simulink model "sim_IDmodel_3pools"  (Simulink 6.3)
settings: Solver=ode45  StartTime=0.0  StopTime=100  RelTol=1e-7
values from neighbouring files (symbols this model uses):
  Ad = [1 5 1]    [PI_mixed_3pools.m]
  dec_DD = 1*[0.8 0.9]    [PI_mixed_3pools.m]
  dec_LU = 1*[1 1]    [PI_mixed_3pools.m]
  t_step1 = 1    [PI_mixed_3pools.m]
  t_step2 = 50    [PI_mixed_3pools.m]
  t_step3 = 100    [PI_mixed_3pools.m]
  tau = [1 1 1]    [PI_mixed_3pools.m]
undefined symbols (not defined in the file or in its folder): K1, K1b, K2
libraries: cstblocks x9
settings Model: LastModifiedBy=IRMOPerm  StrictBusMsg=None
settings DataIOCC: SignalLoggingName=sigsOut
settings DebuggingCC: SolverPrmCheckMsg=none
settings HardwareCC: TargetUnknown=on
settings GRTTargetCC: ModelReferenceCompliant=off  MatFileLogging=off

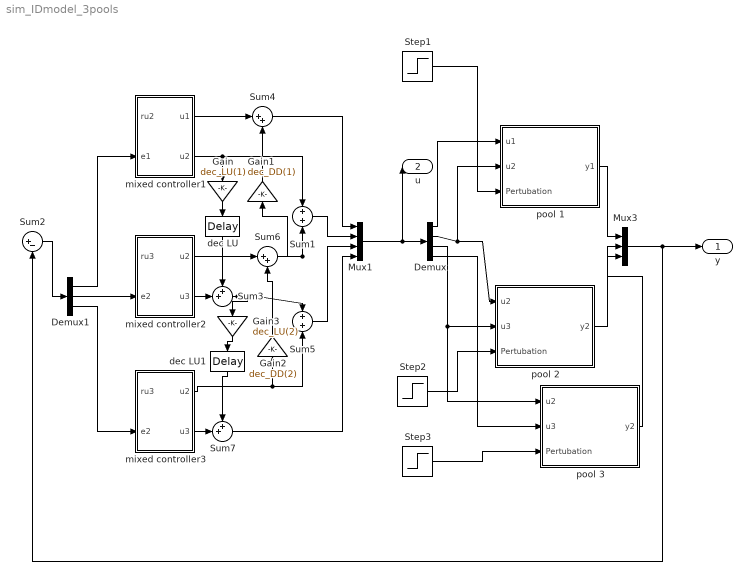
== system sim_IDmodel_3pools ==
  Demux : Demux
  Demux1 : Demux  Outputs=3
  Gain : Gain  Orientation=down  Gain=dec_LU(1)
  Gain1 : Gain  Orientation=up  Gain=dec_DD(1)
  Gain2 : Gain  Orientation=up  Gain=dec_DD(2)
  Gain3 : Gain  Orientation=down  Gain=dec_LU(2)
  Mux1 : Mux
  Mux3 : Mux  Inputs=3
  Step1 : Step  Time=t_step1  SampleTime=0
  Step2 : Step  Time=t_step2  SampleTime=0
  Step3 : Step  Time=t_step3  SampleTime=0
  Sum1 : Sum  SaturateOnIntegerOverflow=on  InputSameDT=on
  Sum2 : Sum  Inputs=|+-  SaturateOnIntegerOverflow=on  InputSameDT=on
  Sum3 : Sum  Inputs=++|  SaturateOnIntegerOverflow=on  InputSameDT=on
  Sum4 : Sum  Inputs=|++  SaturateOnIntegerOverflow=on  InputSameDT=on
  Sum5 : Sum  SaturateOnIntegerOverflow=on  InputSameDT=on
  Sum6 : Sum  Inputs=|++  SaturateOnIntegerOverflow=on  InputSameDT=on
  Sum7 : Sum  Inputs=++|  SaturateOnIntegerOverflow=on  InputSameDT=on
  dec LU : TransportDelay  Orientation=down  DelayTime=tau(2)
  dec LU1 : TransportDelay  Orientation=down  DelayTime=tau(3)
  mixed controller1 : Subsystem
  mixed controller2 : Subsystem
  mixed controller3 : Subsystem
  pool 1 : Subsystem
  pool 2 : Subsystem
  pool 3 : Subsystem
  y : Outport
  u : Outport  Port=2
  wires:
  Mux1/1 -> u/1, Demux/1
  Sum2/1 -> Demux1/1
  Step1/1 -> pool 1/3(Pertubation)
  Demux/2 -> pool 1/2(u2), pool 2/1("u2 ")
  pool 1/1(y1) -> Mux3/1
  pool 2/1(y2) -> Mux3/2
  Demux/1 -> pool 1/1("u1 ")
  Demux/3 -> pool 2/2(u3), pool 3/1("u2 ")
  Mux3/1 -> Sum2/2, y/1
  Demux1/2 -> mixed controller2/2(e2)
  Demux1/1 -> mixed controller1/2(e1)
  mixed controller1/2(u2) -> Sum1/1, Gain/1
  mixed controller2/1(u2) -> Sum6/1
  dec LU/1 -> Sum3/1
  mixed controller2/2(u3) -> Sum3/2
  Gain/1 -> dec LU/1
  Gain1/1 -> Sum4/2
  mixed controller1/1(u1) -> Sum4/1
  Sum4/1 -> Mux1/1
  Sum1/1 -> Mux1/2
  Step2/1 -> pool 2/3(Pertubation)
  Demux1/3 -> mixed controller3/2(e2)
  Sum3/1 -> Gain3/1, Sum5/1
  Gain2/1 -> Sum6/2
  mixed controller3/1(u2) -> Sum5/2, Gain2/1
  dec LU1/1 -> Sum7/1
  Gain3/1 -> dec LU1/1
  Sum7/1 -> Mux1/4
  mixed controller3/2(u3) -> Sum7/2
  Sum6/1 -> Sum1/2, Gain1/1
  Sum5/1 -> Mux1/3
  Demux/4 -> pool 3/2(u3)
  Step3/1 -> pool 3/3(Pertubation)
  pool 3/1(y2) -> Mux3/3

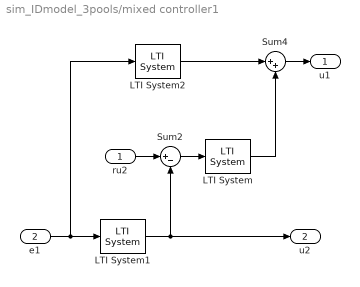
== system sim_IDmodel_3pools/mixed controller1 ==
  ru2 : Inport
  e1 : Inport  Port=2
  LTI System : cstblocks/LTI System  sys=K1b(1)  IC=[]
  LTI System1 : cstblocks/LTI System  sys=K2(1)  IC=[]
  LTI System2 : cstblocks/LTI System  sys=K1(1)  IC=[]
  Sum2 : Sum  Inputs=|+-  SaturateOnIntegerOverflow=on  InputSameDT=on
  Sum4 : Sum  Inputs=|++  SaturateOnIntegerOverflow=on  InputSameDT=on
  u1 : Outport
  u2 : Outport  Port=2
  wires:
  e1/1 -> LTI System2/1, LTI System1/1
  LTI System2/1 -> Sum4/1
  LTI System/1 -> Sum4/2
  Sum2/1 -> LTI System/1
  LTI System1/1 -> Sum2/2, u2/1
  Sum4/1 -> u1/1
  ru2/1 -> Sum2/1

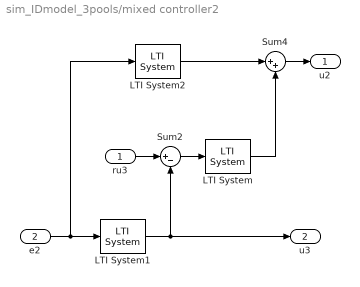
== system sim_IDmodel_3pools/mixed controller2 ==
  ru3 : Inport
  e2 : Inport  Port=2
  LTI System : cstblocks/LTI System  sys=K1b(2)  IC=[]
  LTI System1 : cstblocks/LTI System  sys=K2(2)  IC=[]
  LTI System2 : cstblocks/LTI System  sys=K1(2)  IC=[]
  Sum2 : Sum  Inputs=|+-  SaturateOnIntegerOverflow=on  InputSameDT=on
  Sum4 : Sum  Inputs=|++  SaturateOnIntegerOverflow=on  InputSameDT=on
  u2 : Outport
  u3 : Outport  Port=2
  wires:
  e2/1 -> LTI System2/1, LTI System1/1
  LTI System2/1 -> Sum4/1
  LTI System/1 -> Sum4/2
  Sum2/1 -> LTI System/1
  LTI System1/1 -> Sum2/2, u3/1
  Sum4/1 -> u2/1
  ru3/1 -> Sum2/1

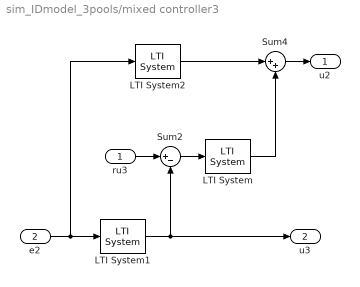
== system sim_IDmodel_3pools/mixed controller3 ==
  ru3 : Inport
  e2 : Inport  Port=2
  LTI System : cstblocks/LTI System  sys=K1b(3)  IC=[]
  LTI System1 : cstblocks/LTI System  sys=K2(3)  IC=[]
  LTI System2 : cstblocks/LTI System  sys=K1(3)  IC=[]
  Sum2 : Sum  Inputs=|+-  SaturateOnIntegerOverflow=on  InputSameDT=on
  Sum4 : Sum  Inputs=|++  SaturateOnIntegerOverflow=on  InputSameDT=on
  u2 : Outport
  u3 : Outport  Port=2
  wires:
  ru3/1 -> Sum2/1
  Sum4/1 -> u2/1
  LTI System1/1 -> u3/1, Sum2/2
  Sum2/1 -> LTI System/1
  LTI System/1 -> Sum4/2
  LTI System2/1 -> Sum4/1
  e2/1 -> LTI System1/1, LTI System2/1

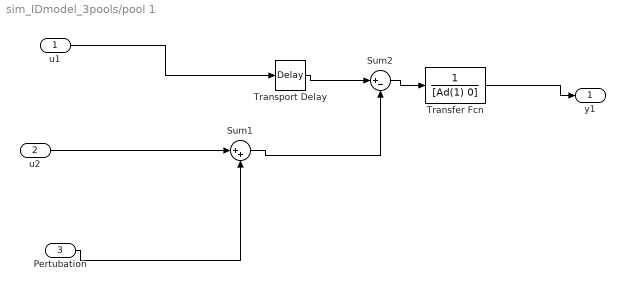
== system sim_IDmodel_3pools/pool 1 ==
  "u1 " : Inport
  u2 : Inport  Port=2
  Pertubation : Inport  Port=3
  Sum1 : Sum  Inputs=|++  SaturateOnIntegerOverflow=on  InputSameDT=on
  Sum2 : Sum  Inputs=|+-  SaturateOnIntegerOverflow=on  InputSameDT=on
  Transfer Fcn : TransferFcn  Denominator=[Ad(1) 0]
  Transport Delay : TransportDelay  DelayTime=tau(1)
  y1 : Outport
  wires:
  Pertubation/1 -> Sum1/2
  Sum1/1 -> Sum2/2
  u2/1 -> Sum1/1
  "u1 "/1 -> Transport Delay/1
  Transport Delay/1 -> Sum2/1
  Sum2/1 -> Transfer Fcn/1
  Transfer Fcn/1 -> y1/1

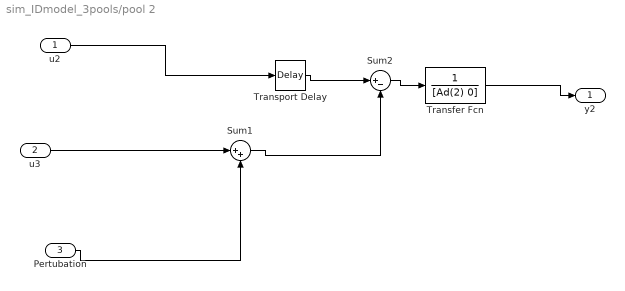
== system sim_IDmodel_3pools/pool 2 ==
  "u2 " : Inport
  u3 : Inport  Port=2
  Pertubation : Inport  Port=3
  Sum1 : Sum  Inputs=|++  SaturateOnIntegerOverflow=on  InputSameDT=on
  Sum2 : Sum  Inputs=|+-  SaturateOnIntegerOverflow=on  InputSameDT=on
  Transfer Fcn : TransferFcn  Denominator=[Ad(2) 0]
  Transport Delay : TransportDelay  DelayTime=tau(2)
  y2 : Outport
  wires:
  Transfer Fcn/1 -> y2/1
  Sum2/1 -> Transfer Fcn/1
  Transport Delay/1 -> Sum2/1
  "u2 "/1 -> Transport Delay/1
  u3/1 -> Sum1/1
  Sum1/1 -> Sum2/2
  Pertubation/1 -> Sum1/2

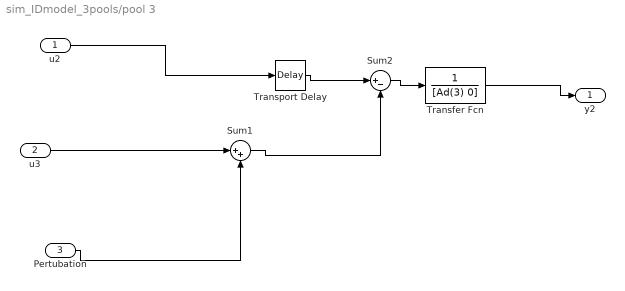
== system sim_IDmodel_3pools/pool 3 ==
  "u2 " : Inport
  u3 : Inport  Port=2
  Pertubation : Inport  Port=3
  Sum1 : Sum  Inputs=|++  SaturateOnIntegerOverflow=on  InputSameDT=on
  Sum2 : Sum  Inputs=|+-  SaturateOnIntegerOverflow=on  InputSameDT=on
  Transfer Fcn : TransferFcn  Denominator=[Ad(3) 0]
  Transport Delay : TransportDelay  DelayTime=tau(3)
  y2 : Outport
  wires:
  Pertubation/1 -> Sum1/2
  Sum1/1 -> Sum2/2
  u3/1 -> Sum1/1
  "u2 "/1 -> Transport Delay/1
  Transport Delay/1 -> Sum2/1
  Sum2/1 -> Transfer Fcn/1
  Transfer Fcn/1 -> y2/1
